simulink model "simulink_02"  (R2017b)
settings: Solver=ode45  StartTime=0.0  StopTime=10.0  RelTol=1e-3
settings Model: Creator=hp  LastModifiedBy=hp

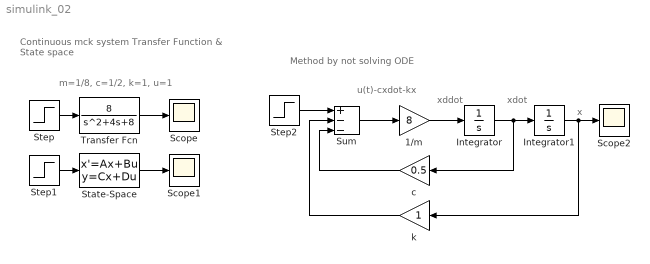
== system simulink_02 ==
  note: u(t)-cxdot-kx
  note: m=1/8, c=1/2, k=1, u=1
  note: Method by not solving ODE
  note: Continuous mck system
      | Transfer Function & State space
  note: xddot
  note: xdot
  note: x
  1/m : Gain  Gain=8
  Integrator : Integrator
  Integrator1 : Integrator
  Scope : Scope
  Scope1 : Scope
  Scope2 : Scope
  State-Space : StateSpace  A=[0 1;-8 -4]  B=[0;8]  C=[1 0]  D=0  InitialCondition=0
  Step : Step  SampleTime=0
  Step1 : Step  SampleTime=0
  Step2 : Step  SampleTime=0
  Sum : Sum  Inputs=+--
  Transfer Fcn : TransferFcn  Numerator=[8]  Denominator=[1 4 8]
  c : Gain  Gain=0.5
  k : Gain
  wires:
  Step/1 -> Transfer Fcn/1
  Transfer Fcn/1 -> Scope/1
  State-Space/1 -> Scope1/1
  Step1/1 -> State-Space/1
  Step2/1 -> Sum/1
  Sum/1 -> 1/m/1
  Integrator/1 -> c/1, Integrator1/1
  1/m/1 -> Integrator/1
  c/1 -> Sum/3
  k/1 -> Sum/2
  Integrator1/1 -> k/1, Scope2/1
